simulink model "one"  (R2016a)
settings: Solver=FixedStepDiscrete  StartTime=0.0  StopTime=10.0  FixedStep=0.01  RelTol=1e-3
libraries: simulink x1
settings Model: Creator=eruffaldi  LastModifiedBy=eruffaldi

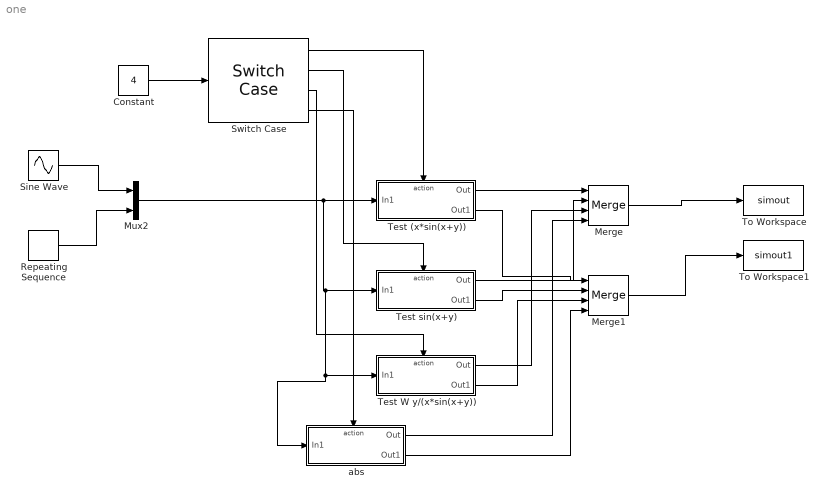
== system one ==
  Constant : Constant  Value=4
  Merge : Merge  Inputs=4
  Merge1 : Merge  Inputs=4
  Mux2 : Mux  Inputs=2
  Repeating Sequence : simulink/Sources/Repeating Sequence  rep_seq_t=[0 2]  rep_seq_y=[0 2]
  Sine Wave : Sin  SampleTime=0
  Switch Case : SwitchCase  CaseConditions={1,2,3,4}  ShowDefaultCase=off
  Test (x*sin(x+y)) : Subsystem  TreatAsAtomicUnit=on
  Test W y/(x*sin(x+y)) : Subsystem  TreatAsAtomicUnit=on
  Test sin(x+y) : Subsystem  TreatAsAtomicUnit=on
  To Workspace : ToWorkspace  VariableName=simout  SaveFormat=Timeseries  SampleTime=-1
  To Workspace1 : ToWorkspace  VariableName=simout1  SaveFormat=Timeseries  SampleTime=-1
  abs : Subsystem  TreatAsAtomicUnit=on
  wires:
  Constant/1 -> Switch Case/1
  Sine Wave/1 -> Mux2/1
  Repeating Sequence/1 -> Mux2/2
  Switch Case/1 -> Test (x*sin(x+y))/Action
  Mux2/1 -> abs/1(In1), Test W y/(x*sin(x+y))/1(In1), Test sin(x+y)/1(In1), Test (x*sin(x+y))/1(In1)
  Switch Case/2 -> Test sin(x+y)/Action
  Merge/1 -> To Workspace/1
  Merge1/1 -> To Workspace1/1
  Switch Case/3 -> Test W y/(x*sin(x+y))/Action
  Switch Case/4 -> abs/Action
  Test (x*sin(x+y))/1(Out) -> Merge/1
  Test sin(x+y)/1(Out) -> Merge/2
  Test W y/(x*sin(x+y))/1(Out) -> Merge/3
  abs/1(Out) -> Merge/4
  Test (x*sin(x+y))/2(Out1) -> Merge1/1
  Test sin(x+y)/2(Out1) -> Merge1/2
  Test W y/(x*sin(x+y))/2(Out1) -> Merge1/3
  abs/2(Out1) -> Merge1/4

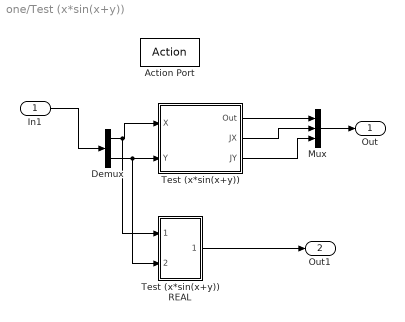
== system one/Test (x*sin(x+y)) ==
  In1 : Inport
  Action Port : ActionPort  ActionType=case
  Demux : Demux  Outputs=2
  Mux : Mux  Inputs=3
  Test (x*sin(x+y)) : Subsystem
  Test (x*sin(x+y)) REAL : Subsystem
  Out : Outport
  Out1 : Outport  Port=2
  wires:
  Demux/2 -> Test (x*sin(x+y)) REAL/2(In2), Test (x*sin(x+y))/2(Y)
  In1/1 -> Demux/1
  Demux/1 -> Test (x*sin(x+y)) REAL/1(In1), Test (x*sin(x+y))/1(X)
  Test (x*sin(x+y))/1(Out) -> Mux/1
  Test (x*sin(x+y))/2(JX) -> Mux/2
  Test (x*sin(x+y))/3(JY) -> Mux/3
  Mux/1 -> Out/1
  Test (x*sin(x+y)) REAL/1(Out1) -> Out1/1

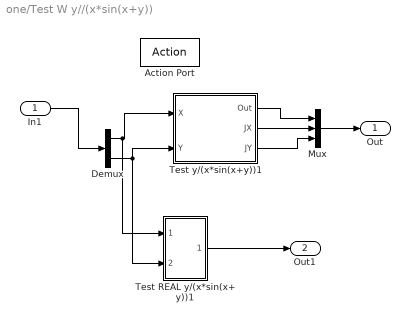
== system one/Test W y//(x*sin(x+y)) ==
  In1 : Inport
  Action Port : ActionPort  ActionType=case
  Demux : Demux  Outputs=2
  Mux : Mux  Inputs=3
  Test REAL y/(x*sin(x+y))1 : Subsystem
  Test y/(x*sin(x+y))1 : Subsystem
  Out : Outport
  Out1 : Outport  Port=2
  wires:
  Demux/2 -> Test y/(x*sin(x+y))1/2(Y), Test REAL y/(x*sin(x+y))1/2(In2)
  In1/1 -> Demux/1
  Demux/1 -> Test y/(x*sin(x+y))1/1(X), Test REAL y/(x*sin(x+y))1/1(In1)
  Test y/(x*sin(x+y))1/1(Out) -> Mux/1
  Test y/(x*sin(x+y))1/2(JX) -> Mux/2
  Test y/(x*sin(x+y))1/3(JY) -> Mux/3
  Mux/1 -> Out/1
  Test REAL y/(x*sin(x+y))1/1(Out1) -> Out1/1

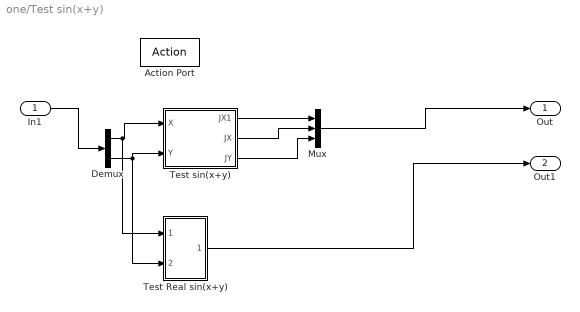
== system one/Test sin(x+y) ==
  In1 : Inport
  Action Port : ActionPort  ActionType=case
  Demux : Demux  Outputs=2
  Mux : Mux  Inputs=3
  Test Real sin(x+y) : Subsystem
  Test sin(x+y) : Subsystem
  Out : Outport
  Out1 : Outport  Port=2
  wires:
  Demux/2 -> Test Real sin(x+y)/2(In2), Test sin(x+y)/2(Y)
  In1/1 -> Demux/1
  Demux/1 -> Test Real sin(x+y)/1(In1), Test sin(x+y)/1(X)
  Test sin(x+y)/1(JX1) -> Mux/1
  Test sin(x+y)/2(JX) -> Mux/2
  Test sin(x+y)/3(JY) -> Mux/3
  Mux/1 -> Out/1
  Test Real sin(x+y)/1(Out1) -> Out1/1

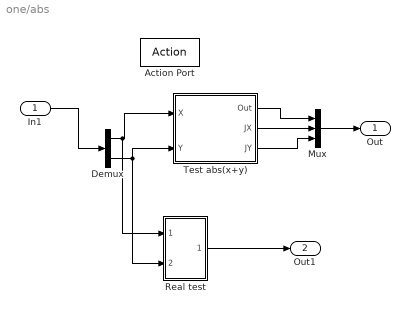
== system one/abs ==
  In1 : Inport
  Action Port : ActionPort  ActionType=case
  Demux : Demux  Outputs=2
  Mux : Mux  Inputs=3
  Real test : Subsystem
  Test abs(x+y) : Subsystem
  Out : Outport
  Out1 : Outport  Port=2
  wires:
  Demux/2 -> Test abs(x+y)/2(Y), Real test/2(In2)
  In1/1 -> Demux/1
  Demux/1 -> Test abs(x+y)/1(X), Real test/1(In1)
  Test abs(x+y)/1(Out) -> Mux/1
  Test abs(x+y)/2(JX) -> Mux/2
  Test abs(x+y)/3(JY) -> Mux/3
  Mux/1 -> Out/1
  Real test/1(Out1) -> Out1/1

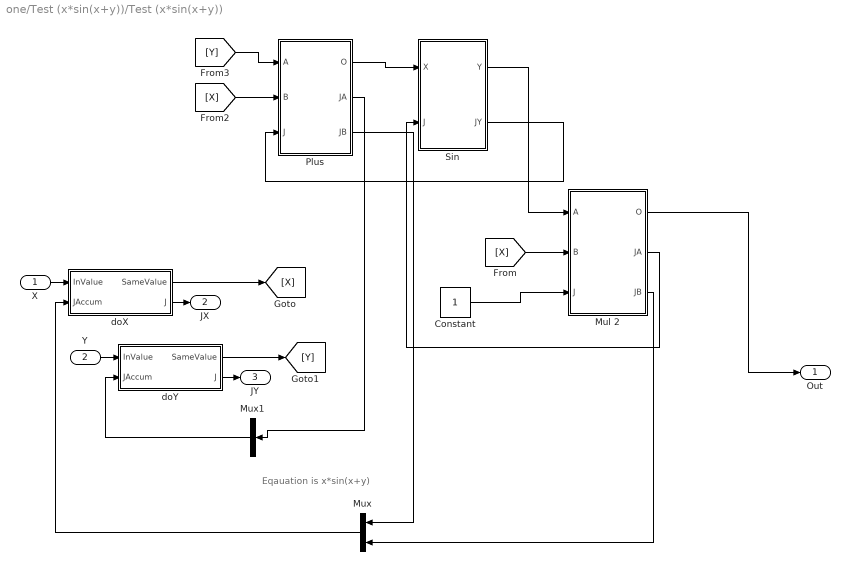
== system one/Test (x*sin(x+y))/Test (x*sin(x+y)) ==
  note: Eqauation is x*sin(x+y)
  X : Inport
  Y : Inport  Port=2
  Constant : Constant
  Mul 2 : Subsystem
  Mux : Mux  Inputs=2
  Mux1 : Mux  Inputs=1
  "Plus " : Subsystem
  Sin : Subsystem
  doX : Subsystem
  doY : Subsystem
  Out : Outport
  JX : Outport  Port=2
  JY : Outport  Port=3
  wires:
  [Y] -> "Plus "/1(A)
  doY/1(SameValue) -> [Y]
  Mux/1 -> doX/2(JAccum)
  "Plus "/1(O) -> Sin/1(X)
  Sin/1(Y) -> Mul 2/1(A)
  Mux1/1 -> doY/2(JAccum)
  Y/1 -> doY/1(InValue)
  "Plus "/3(JB) -> Mux/1
  "Plus "/2(JA) -> Mux1/1
  [X] -> Mul 2/2(B)
  Sin/2(JY) -> "Plus "/3(J)
  doY/2(J) -> JY/1
  Mul 2/3(JB) -> Mux/2
  Mul 2/2(JA) -> Sin/2(J)
  doX/1(SameValue) -> [X]
  doX/2(J) -> JX/1
  X/1 -> doX/1(InValue)
  Mul 2/1(O) -> Out/1
  [X] -> "Plus "/2(B)
  Constant/1 -> Mul 2/3(J)

== system one/Test (x*sin(x+y))/Test (x*sin(x+y)) REAL ==
  In1 : Inport
  In2 : Inport  Port=2
  Fcn3 : Fcn  Expr=u(1)*sin(u(1) + u(2))
  Fcn4 : Fcn  Expr=sin(u(1) + u(2)) + u(1)*cos(u(1) + u(2))
  Fcn5 : Fcn  Expr=u(1)*cos(u(1) + u(2))
  Mux1 : Mux  Inputs=3
  Mux2 : Mux  Inputs=2
  Out1 : Outport
  wires:
  Fcn5/1 -> Mux1/3
  Fcn4/1 -> Mux1/2
  Fcn3/1 -> Mux1/1
  Mux1/1 -> Out1/1
  In1/1 -> Mux2/1
  Mux2/1 -> Fcn5/1, Fcn4/1, Fcn3/1
  In2/1 -> Mux2/2

== system one/Test W y//(x*sin(x+y))/Test REAL y//(x*sin(x+y))1 ==
  In1 : Inport
  In2 : Inport  Port=2
  Fcn3 : Fcn  Expr=u(2)/(u(1)*sin(u(1) + u(2)))
  Fcn4 : Fcn  Expr=-(u(2)*(sin(u(1) + u(2)) + u(1)*cos(u(1) + u(2))))/(u(1)^2*sin(u(1) + u(2))^2)
  Fcn5 : Fcn  Expr=(sin(u(1) + u(2)) - u(2)*cos(u(1) + u(2)))/(u(1)*sin(u(1) + u(2))^2)
  Mux : Mux  Inputs=2
  Mux1 : Mux  Inputs=3
  Out1 : Outport
  wires:
  Fcn5/1 -> Mux1/3
  Fcn4/1 -> Mux1/2
  Fcn3/1 -> Mux1/1
  Mux1/1 -> Out1/1
  Mux/1 -> Fcn5/1, Fcn4/1, Fcn3/1
  In1/1 -> Mux/1
  In2/1 -> Mux/2

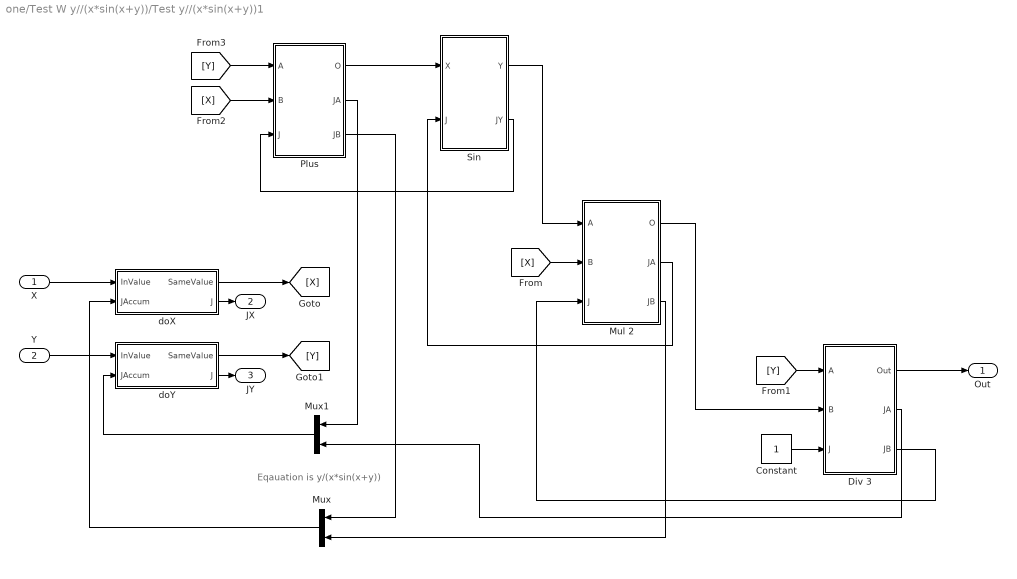
== system one/Test W y//(x*sin(x+y))/Test y//(x*sin(x+y))1 ==
  note: Eqauation is y/(x*sin(x+y))
  X : Inport
  Y : Inport  Port=2
  Constant : Constant
  Div 3 : Subsystem
  Mul 2 : Subsystem
  Mux : Mux  Inputs=2
  Mux1 : Mux  Inputs=2
  "Plus " : Subsystem
  Sin : Subsystem
  doX : Subsystem
  doY : Subsystem
  Out : Outport
  JX : Outport  Port=2
  JY : Outport  Port=3
  wires:
  [Y] -> "Plus "/1(A)
  doY/1(SameValue) -> [Y]
  Mux/1 -> doX/2(JAccum)
  "Plus "/1(O) -> Sin/1(X)
  Sin/1(Y) -> Mul 2/1(A)
  Mux1/1 -> doY/2(JAccum)
  Y/1 -> doY/1(InValue)
  Mul 2/1(O) -> Div 3/2(B)
  "Plus "/3(JB) -> Mux/1
  [Y] -> Div 3/1(A)
  "Plus "/2(JA) -> Mux1/1
  [X] -> Mul 2/2(B)
  Sin/2(JY) -> "Plus "/3(J)
  doY/2(J) -> JY/1
  Mul 2/3(JB) -> Mux/2
  Mul 2/2(JA) -> Sin/2(J)
  doX/1(SameValue) -> [X]
  doX/2(J) -> JX/1
  X/1 -> doX/1(InValue)
  Div 3/1(Out) -> Out/1
  [X] -> "Plus "/2(B)
  Constant/1 -> Div 3/3(J)
  Div 3/3(JB) -> Mul 2/3(J)
  Div 3/2(JA) -> Mux1/2

== system one/Test sin(x+y)/Test Real sin(x+y) ==
  In1 : Inport
  In2 : Inport  Port=2
  Fcn : Fcn  Expr=sin(u(1) + u(2))
  Fcn1 : Fcn  Expr=cos(u(1) + u(2))
  Fcn2 : Fcn  Expr=cos(u(1) + u(2))
  Mux1 : Mux  Inputs=3
  Mux2 : Mux  Inputs=2
  Out1 : Outport
  wires:
  Fcn1/1 -> Mux1/2
  Fcn/1 -> Mux1/1
  Mux1/1 -> Out1/1
  Mux2/1 -> Fcn2/1, Fcn1/1, Fcn/1
  Fcn2/1 -> Mux1/3
  In1/1 -> Mux2/1
  In2/1 -> Mux2/2

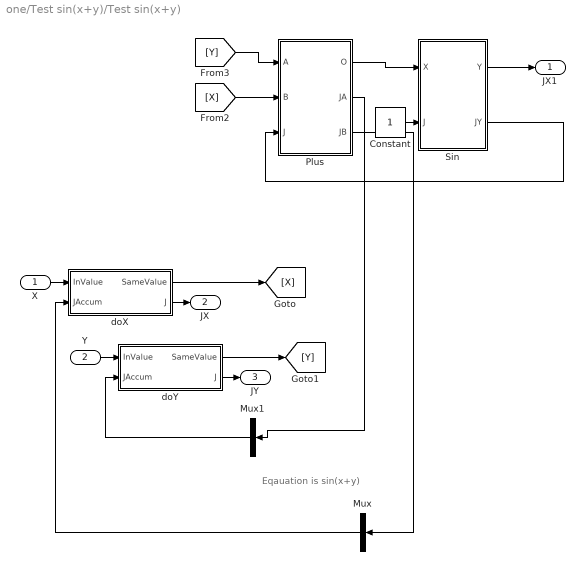
== system one/Test sin(x+y)/Test sin(x+y) ==
  note: Eqauation is sin(x+y)
  X : Inport
  Y : Inport  Port=2
  Constant : Constant
  Mux : Mux  Inputs=1
  Mux1 : Mux  Inputs=1
  "Plus " : Subsystem
  Sin : Subsystem
  doX : Subsystem
  doY : Subsystem
  JX1 : Outport
  JX : Outport  Port=2
  JY : Outport  Port=3
  wires:
  [Y] -> "Plus "/1(A)
  doY/1(SameValue) -> [Y]
  Mux/1 -> doX/2(JAccum)
  "Plus "/1(O) -> Sin/1(X)
  Mux1/1 -> doY/2(JAccum)
  Y/1 -> doY/1(InValue)
  "Plus "/3(JB) -> Mux/1
  "Plus "/2(JA) -> Mux1/1
  Sin/2(JY) -> "Plus "/3(J)
  doY/2(J) -> JY/1
  doX/1(SameValue) -> [X]
  doX/2(J) -> JX/1
  X/1 -> doX/1(InValue)
  [X] -> "Plus "/2(B)
  Sin/1(Y) -> JX1/1
  Constant/1 -> Sin/2(J)

== system one/abs/Real test ==
  In1 : Inport
  In2 : Inport  Port=2
  Fcn3 : Fcn  Expr=abs(u(1)+u(2))
  Fcn4 : Fcn  Expr=u(1)+u(2)
  Mux : Mux  Inputs=2
  Mux1 : Mux  Inputs=3
  Sign : Signum
  Out1 : Outport
  wires:
  Fcn4/1 -> Sign/1
  Fcn3/1 -> Mux1/1
  Mux1/1 -> Out1/1
  Mux/1 -> Fcn4/1, Fcn3/1
  In1/1 -> Mux/1
  In2/1 -> Mux/2
  Sign/1 -> Mux1/2, Mux1/3

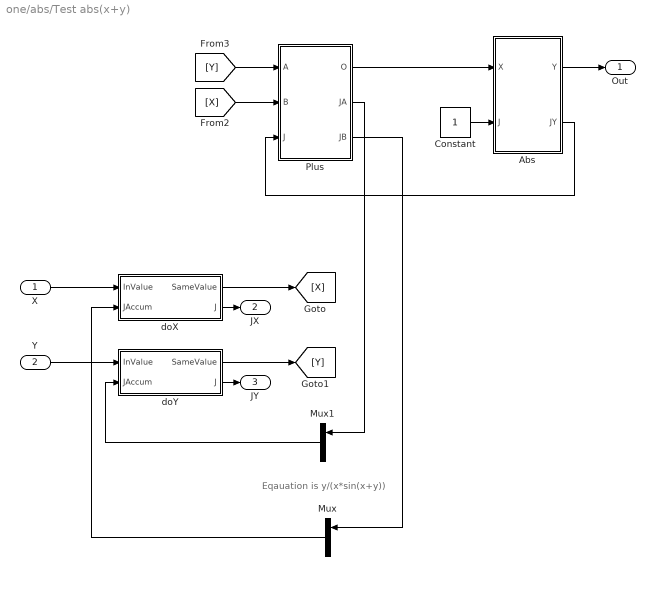
== system one/abs/Test abs(x+y) ==
  note: Eqauation is y/(x*sin(x+y))
  X : Inport
  Y : Inport  Port=2
  Abs : Subsystem
  Constant : Constant
  Mux : Mux  Inputs=2
  Mux1 : Mux  Inputs=2
  "Plus " : Subsystem
  doX : Subsystem
  doY : Subsystem
  Out : Outport
  JX : Outport  Port=2
  JY : Outport  Port=3
  wires:
  [Y] -> "Plus "/1(A)
  doY/1(SameValue) -> [Y]
  Mux/1 -> doX/2(JAccum)
  "Plus "/1(O) -> Abs/1(X)
  Mux1/1 -> doY/2(JAccum)
  Y/1 -> doY/1(InValue)
  "Plus "/3(JB) -> Mux/1
  "Plus "/2(JA) -> Mux1/1
  Abs/2(JY) -> "Plus "/3(J)
  doY/2(J) -> JY/1
  doX/1(SameValue) -> [X]
  doX/2(J) -> JX/1
  X/1 -> doX/1(InValue)
  Abs/1(Y) -> Out/1
  [X] -> "Plus "/2(B)
  Constant/1 -> Abs/2(J)

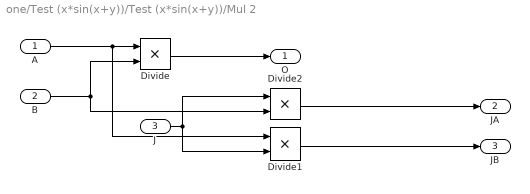
== system one/Test (x*sin(x+y))/Test (x*sin(x+y))/Mul 2 ==
  A : Inport
  B : Inport  Port=2
  J : Inport  Port=3
  Divide : Product  Inputs=**
  Divide1 : Product  Inputs=**
  Divide2 : Product  Inputs=**
  O : Outport
  JA : Outport  Port=2
  JB : Outport  Port=3
  wires:
  Divide/1 -> O/1
  A/1 -> Divide1/1, Divide/1
  Divide1/1 -> JB/1
  Divide2/1 -> JA/1
  B/1 -> Divide2/2, Divide/2
  J/1 -> Divide2/1, Divide1/2

== system one/Test (x*sin(x+y))/Test (x*sin(x+y))/Plus  ==
  A : Inport
  B : Inport  Port=2
  J : Inport  Port=3
  Add : Sum
  O : Outport
  JA : Outport  Port=2
  JB : Outport  Port=3
  wires:
  Add/1 -> O/1
  A/1 -> Add/1
  B/1 -> Add/2
  J/1 -> JB/1, JA/1

== system one/Test (x*sin(x+y))/Test (x*sin(x+y))/Sin ==
  X : Inport
  J : Inport  Port=2
  Product : Product
  Trigonometric Function : Trigonometry
  Trigonometric Function1 : Trigonometry  Operator=cos
  Y : Outport
  JY : Outport  Port=2
  wires:
  Trigonometric Function/1 -> Y/1
  X/1 -> Trigonometric Function1/1, Trigonometric Function/1
  Trigonometric Function1/1 -> Product/1
  J/1 -> Product/2
  Product/1 -> JY/1

== system one/Test (x*sin(x+y))/Test (x*sin(x+y))/doX ==
  InValue : Inport
  JAccum : Inport  Port=2
  Sum of Elements : Sum  Inputs=+
  SameValue : Outport
  J : Outport  Port=2
  wires:
  InValue/1 -> SameValue/1
  JAccum/1 -> Sum of Elements/1
  Sum of Elements/1 -> J/1

== system one/Test (x*sin(x+y))/Test (x*sin(x+y))/doY ==
  InValue : Inport
  JAccum : Inport  Port=2
  Sum of Elements : Sum  Inputs=+
  SameValue : Outport
  J : Outport  Port=2
  wires:
  InValue/1 -> SameValue/1
  JAccum/1 -> Sum of Elements/1
  Sum of Elements/1 -> J/1

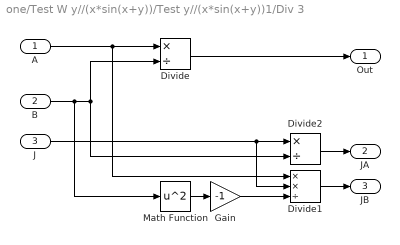
== system one/Test W y//(x*sin(x+y))/Test y//(x*sin(x+y))1/Div 3 ==
  A : Inport
  B : Inport  Port=2
  J : Inport  Port=3
  Divide : Product  Inputs=*/
  Divide1 : Product  Inputs=**/
  Divide2 : Product  Inputs=*/
  Gain : Gain  Gain=-1
  Math Function : Math  Operator=square  SaturateOnIntegerOverflow=on
  Out : Outport
  JA : Outport  Port=2
  JB : Outport  Port=3
  wires:
  Divide/1 -> Out/1
  A/1 -> Divide1/1, Divide/1
  B/1 -> Math Function/1, Divide2/2, Divide/2
  Divide1/1 -> JB/1
  Divide2/1 -> JA/1
  Gain/1 -> Divide1/3
  J/1 -> Divide2/1, Divide1/2
  Math Function/1 -> Gain/1

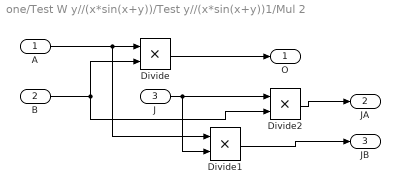
== system one/Test W y//(x*sin(x+y))/Test y//(x*sin(x+y))1/Mul 2 ==
  A : Inport
  B : Inport  Port=2
  J : Inport  Port=3
  Divide : Product  Inputs=**
  Divide1 : Product  Inputs=**
  Divide2 : Product  Inputs=**
  O : Outport
  JA : Outport  Port=2
  JB : Outport  Port=3
  wires:
  Divide/1 -> O/1
  A/1 -> Divide1/1, Divide/1
  Divide1/1 -> JB/1
  Divide2/1 -> JA/1
  B/1 -> Divide2/2, Divide/2
  J/1 -> Divide1/2, Divide2/1

== system one/Test W y//(x*sin(x+y))/Test y//(x*sin(x+y))1/Plus  ==
  A : Inport
  B : Inport  Port=2
  J : Inport  Port=3
  Add : Sum
  O : Outport
  JA : Outport  Port=2
  JB : Outport  Port=3
  wires:
  Add/1 -> O/1
  A/1 -> Add/1
  B/1 -> Add/2
  J/1 -> JB/1, JA/1

== system one/Test W y//(x*sin(x+y))/Test y//(x*sin(x+y))1/Sin ==
  X : Inport
  J : Inport  Port=2
  Product : Product
  Trigonometric Function : Trigonometry
  Trigonometric Function1 : Trigonometry  Operator=cos
  Y : Outport
  JY : Outport  Port=2
  wires:
  Trigonometric Function/1 -> Y/1
  X/1 -> Trigonometric Function1/1, Trigonometric Function/1
  Trigonometric Function1/1 -> Product/1
  J/1 -> Product/2
  Product/1 -> JY/1

== system one/Test W y//(x*sin(x+y))/Test y//(x*sin(x+y))1/doX ==
  InValue : Inport
  JAccum : Inport  Port=2
  Sum of Elements : Sum  Inputs=+
  SameValue : Outport
  J : Outport  Port=2
  wires:
  InValue/1 -> SameValue/1
  JAccum/1 -> Sum of Elements/1
  Sum of Elements/1 -> J/1

== system one/Test W y//(x*sin(x+y))/Test y//(x*sin(x+y))1/doY ==
  InValue : Inport
  JAccum : Inport  Port=2
  Sum of Elements : Sum  Inputs=+
  SameValue : Outport
  J : Outport  Port=2
  wires:
  InValue/1 -> SameValue/1
  JAccum/1 -> Sum of Elements/1
  Sum of Elements/1 -> J/1

== system one/Test sin(x+y)/Test sin(x+y)/Plus  ==
  A : Inport
  B : Inport  Port=2
  J : Inport  Port=3
  Add : Sum
  O : Outport
  JA : Outport  Port=2
  JB : Outport  Port=3
  wires:
  Add/1 -> O/1
  A/1 -> Add/1
  B/1 -> Add/2
  J/1 -> JB/1, JA/1

== system one/Test sin(x+y)/Test sin(x+y)/Sin ==
  X : Inport
  J : Inport  Port=2
  Product : Product
  Trigonometric Function : Trigonometry
  Trigonometric Function1 : Trigonometry  Operator=cos
  Y : Outport
  JY : Outport  Port=2
  wires:
  Trigonometric Function/1 -> Y/1
  X/1 -> Trigonometric Function1/1, Trigonometric Function/1
  Trigonometric Function1/1 -> Product/1
  J/1 -> Product/2
  Product/1 -> JY/1

== system one/Test sin(x+y)/Test sin(x+y)/doX ==
  InValue : Inport
  JAccum : Inport  Port=2
  Sum of Elements : Sum  Inputs=+
  SameValue : Outport
  J : Outport  Port=2
  wires:
  InValue/1 -> SameValue/1
  JAccum/1 -> Sum of Elements/1
  Sum of Elements/1 -> J/1

== system one/Test sin(x+y)/Test sin(x+y)/doY ==
  InValue : Inport
  JAccum : Inport  Port=2
  Sum of Elements : Sum  Inputs=+
  SameValue : Outport
  J : Outport  Port=2
  wires:
  InValue/1 -> SameValue/1
  JAccum/1 -> Sum of Elements/1
  Sum of Elements/1 -> J/1

== system one/abs/Test abs(x+y)/Abs ==
  X : Inport
  J : Inport  Port=2
  Abs : Abs
  Product : Product
  Sign : Signum
  Y : Outport
  JY : Outport  Port=2
  wires:
  Abs/1 -> Y/1
  X/1 -> Sign/1, Abs/1
  Sign/1 -> Product/1
  J/1 -> Product/2
  Product/1 -> JY/1

== system one/abs/Test abs(x+y)/Plus  ==
  A : Inport
  B : Inport  Port=2
  J : Inport  Port=3
  Add : Sum
  O : Outport
  JA : Outport  Port=2
  JB : Outport  Port=3
  wires:
  Add/1 -> O/1
  A/1 -> Add/1
  B/1 -> Add/2
  J/1 -> JB/1, JA/1

== system one/abs/Test abs(x+y)/doX ==
  InValue : Inport
  JAccum : Inport  Port=2
  Sum of Elements : Sum  Inputs=+
  SameValue : Outport
  J : Outport  Port=2
  wires:
  InValue/1 -> SameValue/1
  JAccum/1 -> Sum of Elements/1
  Sum of Elements/1 -> J/1

== system one/abs/Test abs(x+y)/doY ==
  InValue : Inport
  JAccum : Inport  Port=2
  Sum of Elements : Sum  Inputs=+
  SameValue : Outport
  J : Outport  Port=2
  wires:
  InValue/1 -> SameValue/1
  JAccum/1 -> Sum of Elements/1
  Sum of Elements/1 -> J/1
